simulink model "p3B"  (R2018b)
settings: Solver=VariableStepAuto  StartTime=0.0  StopTime=10.0  RelTol=1e-3
libraries: dspsnks4 x1, dspvision x1, dspsigops x1
settings Model: Creator=w_chenxu  LastModifiedBy=valorad

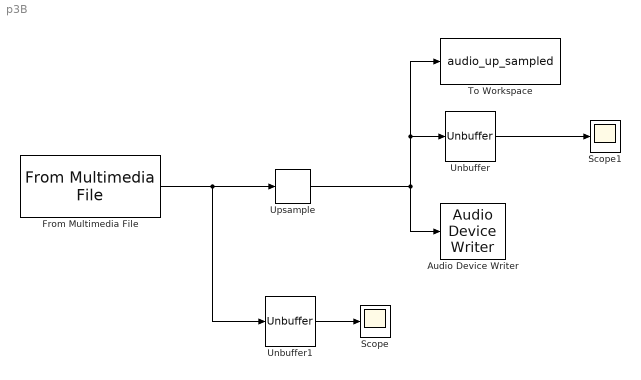
== system p3B ==
  Audio Device Writer : dspsnks4/Audio Device Writer  Driver=ALSA  Device=Default  InheritSampleRate=off  SampleRate=44100  BitDepth=16-bit integer  BufferSize=4096  NumBuffers=10  DefaultOutputChannelMapping=on  OutputChannelMapping=1:2  OutputNumUnderrunSamples=off  DriverIdx=8  DeviceWarnFlag=''
  From Multimedia File : dspvision/From Multimedia File  inputFilename=./musics/ELEC_364_lab_5_Audio_S.wav  loop=on  numPlays=inf  outputStreams=Audio only  videoDataType=single  audioDataType=double  inheritSampleTime=on  userDefinedSampleTime=1/30  noAudioOutput=off  isIntensityVideo=off  fourcc=RGB  colorVideoFormat=One multidimensional signal  outputEOF=off  dataOrg=Column-major  audioFrameSize=1024  computeAudioFrameSize=off  outSamplingMode=Sample based
      settings: SourceProductBaseCode=VP
  Scope : Scope
  Scope1 : Scope
  To Workspace : ToWorkspace  VariableName=audio_up_sampled  SaveFormat=Timeseries  SampleTime=-1
  Unbuffer : Unbuffer
  Unbuffer1 : Unbuffer
  Upsample : dspsigops/Upsample  N=8  phase=0  InputProcessing=Columns as channels (frame based)  RateOptions=Enforce single-rate processing  ic=0  mode=Unused parameter value
  wires:
  Unbuffer/1 -> Scope1/1
  From Multimedia File/1 -> Upsample/1, Unbuffer1/1
  Unbuffer1/1 -> Scope/1
  Upsample/1 -> Audio Device Writer/1, To Workspace/1, Unbuffer/1
